simulink model "Simulation"  (R2023b)
settings: Solver=ode4  StartTime=0.0  StopTime=Te  FixedStep=Ts/20  RelTol=1e-3
undefined symbols (not defined in the file): EgoCar1_params, egoCarID1, targetSpeed, Ts
libraries: drivingscenarioandsensors x7, trackingutilitieslib x2, drivinglib x1, sensorinslib x1
(part 6 of 6)

== matlab function Simulation/Environment/Pack Ego Actor ==
  data: State input; a output Bus: BusActorsActors size=1; ActorID input
function a = packEgo(State, ActorID)
% Pack ego information into a single ego actor bus
%
% Imoprtant note:
% Output is a bus of type BusActorsActors. This is the same bus used by the
% Scenario Reader to output an individual actor. If you change the
% output bus name of Scenario Reader change the output bus name here
% as well by clicking on 'Edit Data' in the menu above.

pos=State.position;
vel=State.velocity;
yaw=State.yaw;
yawRate=State.yawRate;

a = struct(...
    'ActorID',ActorID,...
    'Position', [pos(1) pos(2) 0], ...
    'Velocity', [vel(1) vel(2) 0], ...
    'Roll', 0, ...
    'Pitch', 0, ...
    'Yaw', yaw, ...
    'AngularVelocity', [0 0 yawRate]);
